simulink model "PIDfiltre"  (R2017b)
settings: Solver=FixedStepDiscrete  StartTime=0.0  StopTime=2  FixedStep=Te  RelTol=1e-3  EnableMultiTasking=on
undefined symbols (not defined in the file): DP, DPID, NP, NPID, Te
settings Model: Creator=Avisse  LastModifiedBy=lencs
settings DataIOCC: LimitDataPoints=on  SaveFormat=Array
settings OptimizationCC: LifeSpan=inf
settings DebuggingCC: SolverPrmCheckMsg=warning  SFUnexpectedBacktrackingDiag=warning  SFNoUnconditionalDefaultTransitionDiag=warning  SFExecutionAtInitializationDiag=none
settings HardwareCC: ProdBitPerPointer=32  ProdBitPerSizeT=32  ProdBitPerPtrDiffT=32  ProdLargestAtomicFloat=None  ProdIntDivRoundTo=Undefined  ProdEndianess=Unspecified  ProdWordSize=32  ProdHWDeviceType=32-bit Generic
settings ModelReferenceCC: PropagateSignalLabelsOutOfModel=off
settings CodeAppCC: StateflowObjectComments=on
settings GRTTargetCC: TargetLangStandard=C89/C90 (ANSI)  GeneratePreprocessorConditionals=Disable all
settings ConfigComp: CovMetricSettings=dw  CovHtmlReporting=on  CovSaveCumulativeToWorkspaceVar=on  CovSaveSingleToWorkspaceVar=on  CovExternalEMLEnable=off  CovSFcnEnable=off

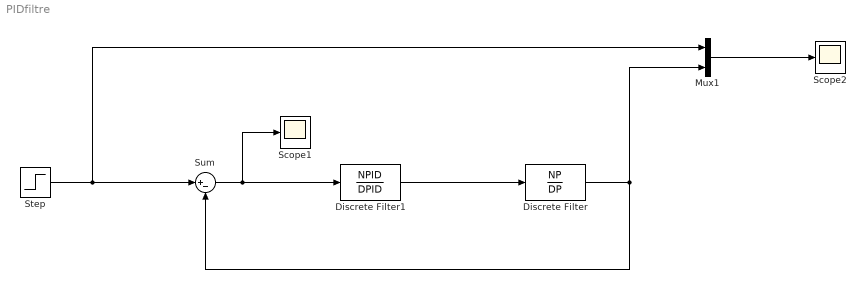
== system PIDfiltre ==
  Discrete Filter : DiscreteFilter  Numerator=NP  Denominator=DP  SampleTime=Te
  Discrete Filter1 : DiscreteFilter  Numerator=NPID  Denominator=DPID  SampleTime=Te
  Mux1 : Mux  Inputs=2
  Scope1 : Scope
  Scope2 : Scope
  Step : Step  SampleTime=0
  Sum : Sum  Inputs=|+-
  wires:
  Step/1 -> Mux1/1, Sum/1
  Discrete Filter/1 -> Sum/2, Mux1/2
  Sum/1 -> Scope1/1, Discrete Filter1/1
  Discrete Filter1/1 -> Discrete Filter/1
  Mux1/1 -> Scope2/1
